simulink library "common_lib"  (R2021b)
settings: Solver=ode45  StartTime=0.0  StopTime=10.0  RelTol=1e-3
undefined symbols (not defined in the file or in its folder): ACCEL_PRE_MULT, C_C1GearNumbers, C_C1GearRatios, C_Calibration, C_DitherWaveform, C_GearOffset, C_GearRatioIn, C_GearRatioInverseOut, C_GearRatioOut, CLUTCH_INNER_LOOP_UPDATE_RATE, CONSTANT, DEGRADED_MODE_SIZE, Dem_EventStatusType, DiscIntNeverNeededParam, F_FAULT_ENUM, F_NOFAULT, F_OUTOFRANGE, F_RATELIMIT, FALSE, FMI14_SPECIAL_INSTRUCTIONS, FMI20_DATA_DRIFTED_HIGH, FMI21_DATA_DRIFTED_LOW, FMI29_RESERVED_FOR_SAE_ASSIGNMENT, FMI30_RESERVED_FOR_SAE_ASSIGNMENT, FMI31_CONDITION_EXISTS, FMI32_NO_FAULT, IC, k_accel, k_mean, LVDCU_OORH_FaultCntThd_C, MAX_UINT32, MEAN_PRE_MULT, NTriggers, QLTY_SIGNAL_FAILED, QLTY_SIGNAL_FULLY_FUNCTION, QLTY_SIGNAL_SUBSTITUTED_BY_1ST_CHOICE, QLTY_SIGNAL_SUBSTITUTED_BY_2ND_CHOICE, QLTY_SIGNAL_SUBSTITUTED_BY_3RD_CHOICE, QLTY_SIGNAL_SUBSTITUTED_BY_4TH_CHOICE, SAMPLE_TIME_100_mSec, SAMPLE_TIME_100_uSec, simin, T_TestPoint, TF_FALSE, TF_TRUE, TimeStep, TRUE, WORKSPACE_UPDATE_RATE, ZERO, Zero
libraries: $bdroot x120, simulink x27, simulink_extras x4, MBD_EPS_Local_Blockset x4
(part 9 of 10)

== system common_lib/Signal Conditioning/HydValveDither/CalculateActualFreq ==
  desired_freqency_hz : Inport
  sample_time : Inport  Port=2
  ClampAroundZero : $bdroot/Misc/ClampAroundZero  Tol=single(eps)
      settings: AttributesFormatString=tol=%<Tol>
  ClampAroundZero1 : $bdroot/Misc/ClampAroundZero  Tol=single(eps)
      settings: AttributesFormatString=tol=%<Tol>
  Constant4 : Constant  Value=single(0)
  Constant7 : Constant  Value=single(1)
  Constant8 : Constant  Value=single(1)
  Product4 : Product  RndMeth=Zero
  Product5 : Product  Inputs=*/  RndMeth=Zero
  Product6 : Product  RndMeth=Zero
  Product7 : Product  Inputs=*/  RndMeth=Zero
  Rounding Function : Rounding  Operator=round
  Switch : Switch  Criteria=u2 > Threshold
  realized_freq : Outport  VectorParamsAs1DForOutWhenUnconnected=off
  sample_times_per_cycle : Outport  Port=2  VectorParamsAs1DForOutWhenUnconnected=off
  wires:
  sample_time/1 -> Product4/1, Product6/1
  Constant7/1 -> Product5/1
  Product5/1 -> Rounding Function/1, sample_times_per_cycle/1  "sample_times_per_period"
  Rounding Function/1 -> Product6/2
  Constant8/1 -> Product7/1
  Product6/1 -> ClampAroundZero1/1
  desired_freqency_hz/1 -> Product4/2, Switch/2
  Product4/1 -> ClampAroundZero/1
  ClampAroundZero/1 -> Product5/2
  ClampAroundZero1/1 -> Product7/2
  Product7/1 -> Switch/1
  Switch/1 -> realized_freq/1
  Constant4/1 -> Switch/3

== system common_lib/Signal Conditioning/HydValveDither/TableBasedSignalGen ==
  sample_times_per_cycle : Inport
  Constant1 : Constant  Value=single(32768)
  Constant5 : Constant  Value=int32(1)
  Constant6 : Constant  Value=length(DitherWaveform)-1  OutDataTypeStr=uint16
  Constant9 : Constant  Value=length(DitherWaveform)-1  OutDataTypeStr=single
  Data Type Conversion2 : DataTypeConversion  OutDataTypeStr=uint16  RndMeth=Nearest
  Data Type Conversion3 : DataTypeConversion  OutDataTypeStr=int32  RndMeth=Nearest
  Direct Lookup Table (n-D) : LookupNDDirect  NumberOfTableDimensions=1  Table=DitherWaveform
  Discrete-Time Integrator : DiscreteIntegrator  IntegratorMethod=Accumulation: Forward Euler  ExternalReset=rising  SampleTime=ts  ShowStatePort=on  ICPrevOutput=DiscIntNeverNeededParam  ICPrevScaledInput=DiscIntNeverNeededParam
  MinMax : MinMax  Inputs=2
  MinMax1 : MinMax  Inputs=2
  Product8 : Product  Inputs=*/*  RndMeth=Zero
  Relational Operator : RelationalOperator  Operator=<=  OutDataTypeStr=boolean  RndMeth=Nearest
  out : Outport  VectorParamsAs1DForOutWhenUnconnected=off
  wires:
  Discrete-Time Integrator/1 -> Product8/1
  Relational Operator/1 -> [reset_integrator]
  [reset_integrator] -> Discrete-Time Integrator/2
  Product8/1 -> Data Type Conversion2/1
  Discrete-Time Integrator/State -> Relational Operator/2
  Constant5/1 -> Discrete-Time Integrator/1
  Data Type Conversion3/1 -> Relational Operator/1
  Constant9/1 -> Product8/3
  Constant6/1 -> MinMax/2
  Data Type Conversion2/1 -> MinMax/1
  MinMax/1 -> Direct Lookup Table (n-D)/1
  Direct Lookup Table (n-D)/1 -> out/1
  sample_times_per_cycle/1 -> Product8/2, MinMax1/2
  MinMax1/1 -> Data Type Conversion3/1
  Constant1/1 -> MinMax1/1

== system common_lib/Signal Conditioning/Obsolete Signal Conditioning/BooleanToTernary ==
  note: Boolean to Ternary Conversion
      | Eaton Corporation
  Boolean : Inport
  Constant1 : Constant  Value=TF_TRUE
  Constant4 : Constant  Value=TF_FALSE
  Switch : Switch  Threshold=0.5  ZeroCross=off
  Ternary : Outport  VectorParamsAs1DForOutWhenUnconnected=off
  wires:
  Boolean/1 -> Switch/2
  Switch/1 -> Ternary/1
  Constant4/1 -> Switch/3
  Constant1/1 -> Switch/1

== system common_lib/Signal Conditioning/Obsolete Signal Conditioning/Ternary To Boolean (Default False) ==
  note: Ternary To Boolean Conversion (Default False)
      | Eaton Corporation
  note: Outputs a FALSE upon an invalid or FALSE input
      | Outputs a TRUE upon a TRUE (149) input
  Ternary : Inport
  Constant1 : Constant  Value=TF_TRUE
  Data Type Conversion : DataTypeConversion  OutDataTypeStr=uint8  RndMeth=Zero
  Relational Operator : RelationalOperator  Operator===  ZeroCross=off  RndMeth=Nearest
  Boolean : Outport  VectorParamsAs1DForOutWhenUnconnected=off
  wires:
  Ternary/1 -> Data Type Conversion/1
  Relational Operator/1 -> Boolean/1
  Constant1/1 -> Relational Operator/1
  Data Type Conversion/1 -> Relational Operator/2

== system common_lib/Signal Conditioning/Obsolete Signal Conditioning/Ternary To Boolean (Default True) ==
  note: Outputs a TRUE upon an invalid or TRUE input
      | Outputs a FALSE upon a FALSE (89) input
  note: Ternary To Boolean Conversion (Default True)
      | Eaton Corporation
  Ternary : Inport
  Constant1 : Constant  Value=TF_FALSE
  Data Type Conversion : DataTypeConversion  OutDataTypeStr=uint8  RndMeth=Zero
  Relational Operator : RelationalOperator  Operator=~=  ZeroCross=off  RndMeth=Nearest
  Boolean : Outport  VectorParamsAs1DForOutWhenUnconnected=off
  wires:
  Data Type Conversion/1 -> Relational Operator/2
  Constant1/1 -> Relational Operator/1
  Relational Operator/1 -> Boolean/1
  Ternary/1 -> Data Type Conversion/1

== system common_lib/Signal Generators/Clu_2_1_3_1_1_1_TestSignalBuilder/TestFrequencyRamp ==
  TestFreqRampStartFreq : Inport
  TestFreqRampEndFreq : Inport  Port=2
  TestFreqRampTime : Inport  Port=3
  TestSignalEnable : Inport  Port=4
  Test_Reset : Inport  Port=5
  ClampAroundZero2 : $bdroot/Misc/ClampAroundZero  Tol=single(eps(1))
      settings: AttributesFormatString=tol=%<Tol>
  Constant1 : Constant  Value=CLUTCH_INNER_LOOP_UPDATE_RATE
  Constant3 : Constant  Value=ZERO
  Constant30 : Constant  Value=ZERO
  Constant4 : Constant  Value=ZERO
  Data Type Conversion : DataTypeConversion  OutDataTypeStr=single  RndMeth=Zero
  Integrator2 : $bdroot/Ctrl/Integrator  TimeStep=CLUTCH_INNER_LOOP_UPDATE_RATE  IC=single(0.0)
  Product6 : Product  Inputs=*/*  InputSameDT=on  OutDataTypeStr=Inherit: Same as first input
  Sum3 : Sum  Inputs=+-|  InputSameDT=on  OutDataTypeStr=Inherit: Same as first input
  Sum5 : Sum  Inputs=|++  InputSameDT=on  OutDataTypeStr=Inherit: Same as first input
  Switch1 : Switch  Threshold=0.5  ZeroCross=off
  TestFreqRampFreq : Outport  InitialOutput=[single(0)]  VectorParamsAs1DForOutWhenUnconnected=off
      settings: AttributesFormatString=InitialOutput=%<InitialOutput>\nOutputWhenDisabled=%<OutputWhenDisabled>
  wires:
  TestFreqRampEndFreq/1 -> Sum3/1, [TgtFreq]
  TestFreqRampStartFreq/1 -> Sum3/2, [InitFreq]
  Sum3/1 -> Product6/1
  TestFreqRampTime/1 -> ClampAroundZero2/1
  Constant30/1 -> Integrator2/4
  [TgtFreq] -> Integrator2/2
  Constant4/1 -> Integrator2/3
  Integrator2/1 -> Sum5/1
  Sum5/1 -> TestFreqRampFreq/1  "TestFreqRampFreq"
  [InitFreq] -> Sum5/2
  Switch1/1 -> Integrator2/1
  Product6/1 -> Switch1/1
  Constant3/1 -> Switch1/3
  ClampAroundZero2/1 -> Product6/2
  TestSignalEnable/1 -> Switch1/2
  Test_Reset/1 -> Integrator2/5
  Constant1/1 -> Data Type Conversion/1
  Data Type Conversion/1 -> Product6/3

== system common_lib/Signal Generators/Clu_2_1_3_1_1_1_TestSignalBuilder/TestOffsetRamp ==
  TestWaveOffsetRampStart : Inport
  TestWaveOffsetRampEnd : Inport  Port=2
  TestWaveOffsetRampTime : Inport  Port=3
  Test_Enable : Inport  Port=4
  Test_Reset : Inport  Port=5
  ClampAroundZero1 : $bdroot/Misc/ClampAroundZero  Tol=single(eps(1))
      settings: AttributesFormatString=tol=%<Tol>
  Constant11 : Constant  Value=ZERO
  Constant8 : Constant  Value=ZERO
  Constant9 : Constant  Value=ZERO
  Integrator3 : $bdroot/Ctrl/Integrator  TimeStep=CLUTCH_INNER_LOOP_UPDATE_RATE  IC=single(0.0)
  Product4 : Product  Inputs=*/  InputSameDT=on  OutDataTypeStr=Inherit: Same as first input
  Sum7 : Sum  Inputs=+-|  InputSameDT=on  OutDataTypeStr=Inherit: Same as first input
  Switch3 : Switch  Threshold=0.5  ZeroCross=off
  TestConstant : Outport  InitialOutput=[single(0)]  VectorParamsAs1DForOutWhenUnconnected=off
      settings: AttributesFormatString=InitialOutput=%<InitialOutput>\nOutputWhenDisabled=%<OutputWhenDisabled>
  TestOffsetRamp : Outport  Port=2  InitialOutput=[single(0)]  VectorParamsAs1DForOutWhenUnconnected=off
      settings: AttributesFormatString=InitialOutput=%<InitialOutput>\nOutputWhenDisabled=%<OutputWhenDisabled>
  wires:
  TestWaveOffsetRampStart/1 -> Sum7/2
  Sum7/1 -> Product4/1
  TestWaveOffsetRampTime/1 -> ClampAroundZero1/1
  Constant9/1 -> Integrator3/4
  [TestWaveOffsetRampEnd] -> Integrator3/2
  Constant11/1 -> Integrator3/3
  Switch3/1 -> Integrator3/1
  Product4/1 -> Switch3/1
  Constant8/1 -> Switch3/3
  ClampAroundZero1/1 -> Product4/2
  Integrator3/1 -> TestOffsetRamp/1
  TestWaveOffsetRampEnd/1 -> Sum7/1, [TestWaveOffsetRampEnd], TestConstant/1
  Test_Enable/1 -> Switch3/2
  Test_Reset/1 -> Integrator3/5

== system common_lib/Signal Generators/Clu_2_1_3_1_1_1_TestSignalBuilder/TestRampWaves ==
  TestOffsetRamp : Inport
  TestWave : Inport  Port=2
  TestWaveSignSwitch : Inport  Port=3
  Constant : Constant  Value=single(0.0)  SampleTime=-1
  EdgeTriggered Pulse : $bdroot/Misc/EdgeTriggered Pulse  Edge=FALSE to TRUE  Width=single(CLUTCH_INNER_LOOP_UPDATE_RATE)  Pulse=TRUE  TimeStep=CLUTCH_INNER_LOOP_UPDATE_RATE  Init=0
  Hold : $bdroot/Misc/Hold  SystemSampleTime=-1  VariantActivationTime=update diagram  Latency=0  AutoFrameSizeCalculation=off
  Relational Operator : RelationalOperator  Operator=>  ZeroCross=off  RndMeth=Nearest
  Sum1 : Sum  InputSameDT=on  OutDataTypeStr=Inherit: Same as first input
  Sum2 : Sum  InputSameDT=on  OutDataTypeStr=Inherit: Same as first input
  SineWave : Outport  VectorParamsAs1DForOutWhenUnconnected=off
  SquareWave : Outport  Port=2  VectorParamsAs1DForOutWhenUnconnected=off
  wires:
  Sum1/1 -> SineWave/1
  TestOffsetRamp/1 -> Hold/1, Sum1/1
  TestWave/1 -> Sum1/2, Sum2/2
  TestWaveSignSwitch/1 -> Relational Operator/1
  EdgeTriggered Pulse/1 -> Hold/Enable
  Hold/1 -> Sum2/1
  Sum2/1 -> SquareWave/1
  Relational Operator/1 -> EdgeTriggered Pulse/1
  Constant/1 -> Relational Operator/2

== system common_lib/Signal Generators/Clu_2_1_3_1_1_1_TestSignalBuilder/TestWaveCreation ==
  note: Outputtype
      | 0. Constant
      | 1. Ramp
      | 2. Sine Wave
      | 3. Square Wave
      | 4. Zero
  TestFreqRampFreq : Inport
  TestWaveAmplitude : Inport  Port=2
  Test_Reset : Inport  Port=3
  CluPresCmdTestSignalType : Inport  Port=4
  Constant1 : Constant  Value=-1
  Constant10 : Constant  Value=pi/2.0
  Constant12 : Constant  Value=-1.0
  Constant13 : Constant  Value=1.0
  Constant2 : Constant  Value=single(0.0)
  Constant3 : Constant  Value=single(0.0)
  Constant30 : Constant  Value=ZERO
  Constant4 : Constant  Value=single(0.0)
  Data Type Conversion{12..13,19..20} (4 alike) : DataTypeConversion  OutDataTypeStr=single  RndMeth=Zero
  Integrator1 : $bdroot/Ctrl/Integrator  TimeStep=CLUTCH_INNER_LOOP_UPDATE_RATE  IC=single(0.0)
  Multiport Switch : MultiPortSwitch  DataPortOrder=Zero-based contiguous  Inputs=4  DataPortForDefault=Additional data port  zeroidx=on
  Product1 : Product  Inputs=**  InputSameDT=on  OutDataTypeStr=Inherit: Same as first input
  Product2 : Product  Inputs=**  InputSameDT=on  OutDataTypeStr=Inherit: Same as first input
  Product5 : Product  Inputs=**  InputSameDT=on  OutDataTypeStr=Inherit: Same as first input
  Relay : $bdroot/Slink/Relay  init=single(1.0)
  Sine1 : $bdroot/Misc/Sine
  Unit Delay4 : UnitDelay  InitialCondition=single(1.0)  SampleTime=-1  HasFrameUpgradeWarning=on
      settings: AttributesFormatString=ic=%<X0>
  TestWave : Outport  InitialOutput=[single(0)]  VectorParamsAs1DForOutWhenUnconnected=off
      settings: AttributesFormatString=InitialOutput=%<InitialOutput>\nOutputWhenDisabled=%<OutputWhenDisabled>
  TestWaveSignSwitch : Outport  Port=2  InitialOutput=[single(0)]  VectorParamsAs1DForOutWhenUnconnected=off
      settings: AttributesFormatString=InitialOutput=%<InitialOutput>\nOutputWhenDisabled=%<OutputWhenDisabled>
  wires:
  Constant12/1 -> Data Type Conversion19/1
  Constant13/1 -> Data Type Conversion20/1
  Data Type Conversion19/1 -> Relay/4
  Data Type Conversion20/1 -> Relay/5
  Relay/1 -> Unit Delay4/1, Multiport Switch/5, TestWaveSignSwitch/1
  Unit Delay4/1 -> [TestWaveSignSwitch]
  Integrator1/1 -> Relay/1, Sine1/1
  TestWaveAmplitude/1 -> Product2/1
  Product2/1 -> TestWave/1
  [TestWaveSignSwitch] -> Product5/2
  Product5/1 -> Integrator1/1  "ChirpFrequency"
  Constant10/1 -> Data Type Conversion12/1, Product1/1
  Product1/1 -> Data Type Conversion13/1
  Constant1/1 -> Product1/2
  Data Type Conversion12/1 -> Integrator1/2, Relay/2
  Data Type Conversion13/1 -> Integrator1/3, Relay/3
  Constant30/1 -> Integrator1/4
  Test_Reset/1 -> Integrator1/5
  TestFreqRampFreq/1 -> Product5/1
  CluPresCmdTestSignalType/1 -> Multiport Switch/1
  Constant2/1 -> Multiport Switch/2
  Constant3/1 -> Multiport Switch/3
  Constant4/1 -> Multiport Switch/6
  Multiport Switch/1 -> Product2/2
  Sine1/1 -> Multiport Switch/4

== system common_lib/Signal Generators/Signal Generator Components/TestSignalPeriod ==
  TestSignalFrequency : Inport
  ClampAboveZero : $bdroot/Misc/ClampAboveZero  Tol=single(0.0001)
      settings: AttributesFormatString=tol=%<Tol>
  ClampAroundZero1 : $bdroot/Misc/ClampAroundZero  Tol=single(0.01)
      settings: AttributesFormatString=tol=%<Tol>
  Constant1 : Constant  Value=TimeStep  SampleTime=-1
  Constant35 : Constant  Value=single(2.0)  SampleTime=-1
  Constant39 : Constant  Value=single(1.0)  SampleTime=-1
  Data Type Conversion1 : DataTypeConversion  OutDataTypeStr=single
  MinMax1 : MinMax  Function=max  Inputs=2  InputSameDT=on  ZeroCross=off
  Product15 : Product  Inputs=*/  OutDataTypeStr=Inherit: Same as first input
  Product19 : Product  Inputs=**  InputSameDT=on  OutDataTypeStr=Inherit: Same as first input
  TestSignalPeriod : Outport  VectorParamsAs1DForOutWhenUnconnected=off
  wires:
  Product15/1 -> MinMax1/1
  Constant39/1 -> Product15/1
  ClampAroundZero1/1 -> Product15/2
  TestSignalFrequency/1 -> ClampAroundZero1/1
  Constant1/1 -> Data Type Conversion1/1
  Constant35/1 -> Product19/2
  Product19/1 -> MinMax1/2
  MinMax1/1 -> TestSignalPeriod/1  "TestSignalPeriod"
  ClampAboveZero/1 -> Product19/1
  Data Type Conversion1/1 -> ClampAboveZero/1

== system common_lib/Signal Generators/Signal Generator Components/TestSignalPeriodTimer ==
  TestSignalReset : Inport
  TestSignalPeriod : Inport  Port=2
  ClampAboveZero : $bdroot/Misc/ClampAboveZero  Tol=single(0.0001)
      settings: AttributesFormatString=tol=%<Tol>
  Constant1 : Constant  Value=TimeStep  SampleTime=-1
  Constant40 : Constant  Value=false  SampleTime=-1
  Constant41 : Constant  Value=single(0.0)
  Data Type Conversion7 : DataTypeConversion  OutDataTypeStr=single
  Logical Operator1 : Logic  Operator=OR  Inputs=3  AllPortsSameDT=off
  Relational Operator4 : RelationalOperator  ZeroCross=off  RndMeth=Nearest
  Sum5 : Sum  Inputs=2
  Switch5 : Switch  Threshold=0.5  ZeroCross=off
  Unit Delay4 : UnitDelay  InitialCondition=true  SampleTime=-1  HasFrameUpgradeWarning=on
      settings: AttributesFormatString=ic=%<X0>
  Unit Delay5 : UnitDelay  InitialCondition=single(0.0)  SampleTime=-1  HasFrameUpgradeWarning=on
      settings: AttributesFormatString=ic=%<X0>
  TestSignalTime : Outport  VectorParamsAs1DForOutWhenUnconnected=off
  wires:
  TestSignalReset/1 -> Logical Operator1/2
  Logical Operator1/1 -> Switch5/2
  Switch5/1 -> Unit Delay5/1, TestSignalTime/1  "TestSignalTime"
  Sum5/1 -> Switch5/3
  Constant41/1 -> Switch5/1
  Unit Delay4/1 -> Logical Operator1/1
  Constant40/1 -> Unit Delay4/1
  TestSignalPeriod/1 -> Relational Operator4/2
  Relational Operator4/1 -> Logical Operator1/3
  Unit Delay5/1 -> Relational Operator4/1, Sum5/1
  Constant1/1 -> Data Type Conversion7/1
  Data Type Conversion7/1 -> ClampAboveZero/1
  ClampAboveZero/1 -> Sum5/2

== system common_lib/Signal Generators/Signal Generator Components/TestSignalRamp ==
  TestSignalRampStart : Inport
  TestSignalRampEnd : Inport  Port=2
  TestSignalRampTime : Inport  Port=3
  TestSignalReset : Inport  Port=4
  Abs : Abs  ZeroCross=off
  Constant35 : Constant  Value=single(0.01)  SampleTime=-1
  Logical Operator : Logic  AllPortsSameDT=off
  Logical Operator1 : Logic  Operator=NOT  AllPortsSameDT=off
  Logical Operator2 : Logic  Operator=NOT  AllPortsSameDT=off
  Logical Operator3 : Logic  Operator=OR  AllPortsSameDT=off
  Relational Operator : RelationalOperator  ZeroCross=off  RndMeth=Nearest
  Sum : Sum  Inputs=+-
  TestSignalRampEnabled : Subsystem
  Unit Delay : UnitDelay  InitialCondition=CLUTCH_INNER_LOOP_UPDATE_RATE  SampleTime=-1  HasFrameUpgradeWarning=on
      settings: AttributesFormatString=ic=%<X0>
  TestSignal : Outport  VectorParamsAs1DForOutWhenUnconnected=off
  wires:
  Logical Operator3/1 -> Logical Operator/2
  Logical Operator2/1 -> Logical Operator3/2
  Unit Delay/1 -> Logical Operator2/1
  Logical Operator1/1 -> Logical Operator3/1
  Logical Operator/1 -> TestSignalRampEnabled/Enable
  Relational Operator/1 -> Logical Operator/1
  Constant35/1 -> Relational Operator/2
  Abs/1 -> Relational Operator/1
  Sum/1 -> Abs/1
  TestSignalRampTime/1 -> TestSignalRampEnabled/3(TestSignalFreqRampTime)
  TestSignalRampEnabled/1(TestSignalFrequency) -> TestSignal/1
  TestSignalRampEnd/1 -> Sum/2, TestSignalRampEnabled/2(TestSignalFreqRampEnd)
  TestSignalRampStart/1 -> Sum/1, TestSignalRampEnabled/1(TestSignalFrequencyIn)
  TestSignalReset/1 -> Unit Delay/1, Logical Operator1/1, TestSignalRampEnabled/4(TestSignalReset)

== system common_lib/Signal Generators/Signal Generator Components/TestSignalSineWave ==
  TestSignalPk2PkAmplitude : Inport
  TestSignalOffset : Inport  Port=2
  TestSignalTime : Inport  Port=3
  TestSignalPeriod : Inport  Port=4
  TestSignalReset : Inport  Port=5
  Constant1 : Constant  Value=single(0.0)
  Data Type Conversion4 : DataTypeConversion  OutDataTypeStr=uint32  RndMeth=Zero
  Look-Up Table : Lookup  InputValues=single([0 0.25 0.5 0.75 1])  Table=single([0 pi/2 0 -pi/2 0])  LookUpMeth=Interpolation-Use End Values
      settings: AttributesFormatString=X=%<InputValues>\nY= %<OutputValues>
  Product1 : Product  Inputs=*/  OutDataTypeStr=Inherit: Same as first input
  Product16 : Product  Inputs=*/  OutDataTypeStr=Inherit: Same as first input
  Product18 : Product  Inputs=**  OutDataTypeStr=Inherit: Same as first input
  Sine1 : $bdroot/Misc/Sine
  Sum3 : Sum  Inputs=+-
  Sum4 : Sum
  Switch1 : Switch  Threshold=0.5  ZeroCross=off
  TestSignal : Outport  VectorParamsAs1DForOutWhenUnconnected=off
  wires:
  Sine1/1 -> Product18/1
  Look-Up Table/1 -> Sine1/1
  Product1/1 -> Look-Up Table/1  "TestSignalPeriodFrac"
  [TestSignalPeriod] -> Product1/2
  Switch1/1 -> Sum4/1
  Constant1/1 -> Switch1/1
  TestSignalReset/1 -> Switch1/2
  TestSignalPk2PkAmplitude/1 -> Product18/2
  TestSignalOffset/1 -> Sum4/2
  Sum4/1 -> TestSignal/1  "TestSignal"
  Product16/1 -> Sum3/1, Data Type Conversion4/1
  Data Type Conversion4/1 -> Sum3/2
  Sum3/1 -> Product1/1
  Product18/1 -> Switch1/3
  TestSignalTime/1 -> Product16/1, [TestSignalTime]
  TestSignalPeriod/1 -> Product16/2, [TestSignalPeriod]

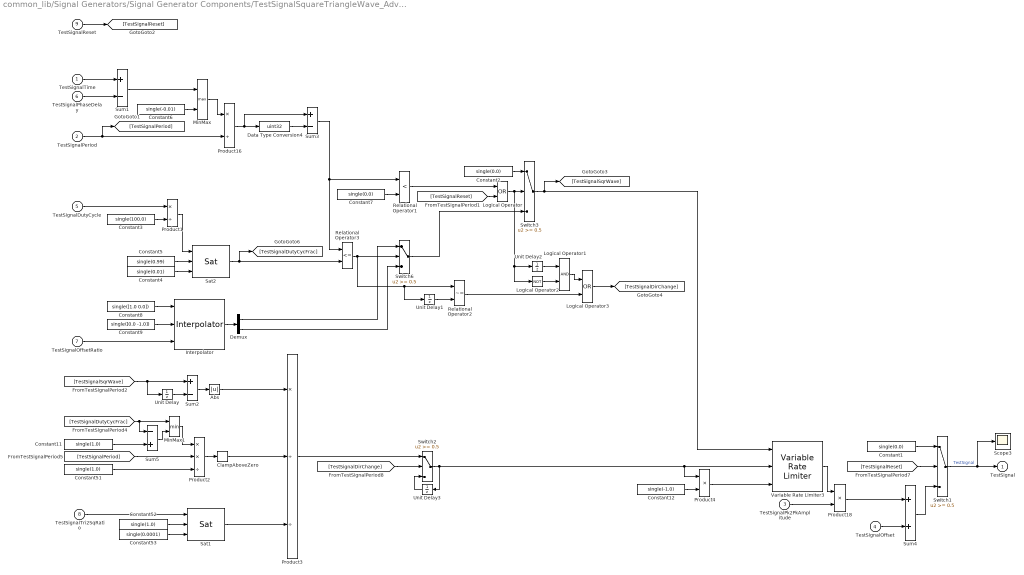
== system common_lib/Signal Generators/Signal Generator Components/TestSignalSquareTriangleWave_Advanced ==
  TestSignalTime : Inport
  TestSignalPeriod : Inport  Port=2
  TestSignalPk2PkAmplitude : Inport  Port=3
  TestSignalOffset : Inport  Port=4
  TestSignalDutyCycle : Inport  Port=5
  TestSignalPhaseDelay : Inport  Port=6
  TestSignalOffsetRatio : Inport  Port=7
  TestSignalTri2SqRatio : Inport  Port=8
  TestSignalReset : Inport  Port=9
  Abs : Abs  ZeroCross=off
  ClampAboveZero : $bdroot/Misc/ClampAboveZero  Tol=single(0.001)
      settings: AttributesFormatString=tol=%<Tol>
  Constant1 : Constant  Value=single(0.0)
  Constant11 : Constant  Value=single(1.0)
  Constant12 : Constant  Value=single(-1.0)
  Constant2 : Constant  Value=single(0.0)
  Constant3 : Constant  Value=single(100.0)
  Constant4 : Constant  Value=single(0.01)
  Constant5 : Constant  Value=single(0.99)
  Constant51 : Constant  Value=single(1.0)
  Constant52 : Constant  Value=single(1.0)
  Constant53 : Constant  Value=single(0.0001)
  Constant6 : Constant  Value=single(-0.01)
  Constant7 : Constant  Value=single(0.0)
  Constant8 : Constant  Value=single([1.0 0.0])
  Constant9 : Constant  Value=single([0.0 -1.0])
  Data Type Conversion4 : DataTypeConversion  OutDataTypeStr=uint32  RndMeth=Zero
  Demux : Demux  Outputs=2
  Interpolator : $bdroot/Tbl/Interpolator  DType=Single
  Logical Operator : Logic  Operator=OR  AllPortsSameDT=off
  Logical Operator1 : Logic  AllPortsSameDT=off
  Logical Operator2 : Logic  Operator=NOT  AllPortsSameDT=off
  Logical Operator3 : Logic  Operator=OR  AllPortsSameDT=off
  MinMax : MinMax  Function=max  Inputs=2  InputSameDT=on  ZeroCross=off
  MinMax1 : MinMax  Inputs=2  InputSameDT=on  ZeroCross=off
  Product1 : Product  Inputs=*/  OutDataTypeStr=Inherit: Same as first input
  Product16 : Product  Inputs=*/  OutDataTypeStr=Inherit: Same as first input
  Product18 : Product  Inputs=**  OutDataTypeStr=Inherit: Same as first input
  Product2 : Product  Inputs=**/  OutDataTypeStr=Inherit: Same as first input
  Product3 : Product  Inputs=*//  OutDataTypeStr=Inherit: Same as first input
  Product4 : Product  Inputs=**  OutDataTypeStr=Inherit: Same as first input
  Relational Operator1 : RelationalOperator  Operator=<  ZeroCross=off  RndMeth=Nearest
  Relational Operator2 : RelationalOperator  Operator=~=  ZeroCross=off  RndMeth=Nearest
  Relational Operator3 : RelationalOperator  Operator=<=  ZeroCross=off  RndMeth=Nearest
  Sat1 : $bdroot/Slink/Sat
  Sat2 : $bdroot/Slink/Sat
  Scope3 : Scope
  Sum1 : Sum  Inputs=+-
  Sum2 : Sum  Inputs=+-
  Sum3 : Sum  Inputs=+-
  Sum4 : Sum
  Sum5 : Sum  Inputs=-+
  Switch{1..3,6} (4 alike) : Switch  Threshold=0.5  ZeroCross=off
  Unit Delay : UnitDelay  InitialCondition=single(0.0)  SampleTime=-1  HasFrameUpgradeWarning=on
      settings: AttributesFormatString=ic=%<X0>
  Unit Delay1 : UnitDelay  InitialCondition=false  SampleTime=-1  HasFrameUpgradeWarning=on
      settings: AttributesFormatString=ic=%<X0>
  Unit Delay2 : UnitDelay  InitialCondition=false  SampleTime=-1  HasFrameUpgradeWarning=on
      settings: AttributesFormatString=ic=%<X0>
  Unit Delay3 : UnitDelay  InitialCondition=single(0.0)  SampleTime=-1  HasFrameUpgradeWarning=on
      settings: AttributesFormatString=ic=%<X0>
  Variable Rate Limiter3 : $bdroot/Slink/Variable Rate Limiter  TimeStep=TimeStep  ic=single(0.0)
  TestSignal : Outport  VectorParamsAs1DForOutWhenUnconnected=off
  wires:
  MinMax1/1 -> Product2/1
  Product4/1 -> Variable Rate Limiter3/3
  Constant12/1 -> Product4/2
  Abs/1 -> Product3/1
  [TestSignalDirChange] -> Switch2/2
  Unit Delay3/1 -> Switch2/3
  Switch2/1 -> Unit Delay3/1, Product4/1, Variable Rate Limiter3/2
  [TestSignalReset] -> Switch1/2
  Product3/1 -> Switch2/1
  Sum5/1 -> MinMax1/2
  Constant11/1 -> Sum5/2
  ClampAboveZero/1 -> Product3/2
  Sum2/1 -> Abs/1
  Product2/1 -> ClampAboveZero/1
  [TestSignalPeriod] -> Product2/2
  [TestSignalDutyCycFrac] -> MinMax1/1, Sum5/1
  Unit Delay/1 -> Sum2/2
  Logical Operator3/1 -> [TestSignalDirChange]
  Relational Operator2/1 -> Logical Operator3/2
  Logical Operator1/1 -> Logical Operator3/1
  Logical Operator2/1 -> Logical Operator1/2
  Unit Delay2/1 -> Logical Operator1/1
  Unit Delay1/1 -> Relational Operator2/2
  [TestSignalSqrWave] -> Sum2/1, Unit Delay/1
  Logical Operator/1 -> Logical Operator2/1, Unit Delay2/1, Switch3/2
  [TestSignalReset] -> Logical Operator/2
  Demux/2 -> Switch6/3
  Demux/1 -> Switch6/1
  Interpolator/1 -> Demux/1
  Constant2/1 -> Switch3/1
  Constant8/1 -> Interpolator/1
  Switch3/1 -> [TestSignalSqrWave], Variable Rate Limiter3/1
  Constant9/1 -> Interpolator/2
  TestSignalOffsetRatio/1 -> Interpolator/3
  Relational Operator1/1 -> Logical Operator/1
  Constant7/1 -> Relational Operator1/2
  MinMax/1 -> Product16/1
  Constant6/1 -> MinMax/2
  TestSignalPhaseDelay/1 -> Sum1/2
  Sum1/1 -> MinMax/1
  Sat2/1 -> [TestSignalDutyCycFrac], Relational Operator3/2
  Constant5/1 -> Sat2/2
  Constant4/1 -> Sat2/3
  Product1/1 -> Sat2/1
  Constant3/1 -> Product1/2
  TestSignalDutyCycle/1 -> Product1/1
  Switch1/1 -> Scope3/1, TestSignal/1  "TestSignal"
  Constant1/1 -> Switch1/1
  Sat1/1 -> Product3/3
  Constant53/1 -> Sat1/3
  Constant52/1 -> Sat1/2
  TestSignalTri2SqRatio/1 -> Sat1/1
  Constant51/1 -> Product2/3
  Variable Rate Limiter3/1 -> Product18/1
  TestSignalPk2PkAmplitude/1 -> Product18/2
  TestSignalOffset/1 -> Sum4/2
  Product16/1 -> Sum3/1, Data Type Conversion4/1
  Data Type Conversion4/1 -> Sum3/2
  Sum3/1 -> Relational Operator1/1, Relational Operator3/1
  Relational Operator3/1 -> Unit Delay1/1, Relational Operator2/1, Switch6/2
  Switch6/1 -> Switch3/3
  Product18/1 -> Sum4/1
  TestSignalTime/1 -> Sum1/1
  TestSignalPeriod/1 -> Product16/2, [TestSignalPeriod]
  Sum4/1 -> Switch1/3
  TestSignalReset/1 -> [TestSignalReset]

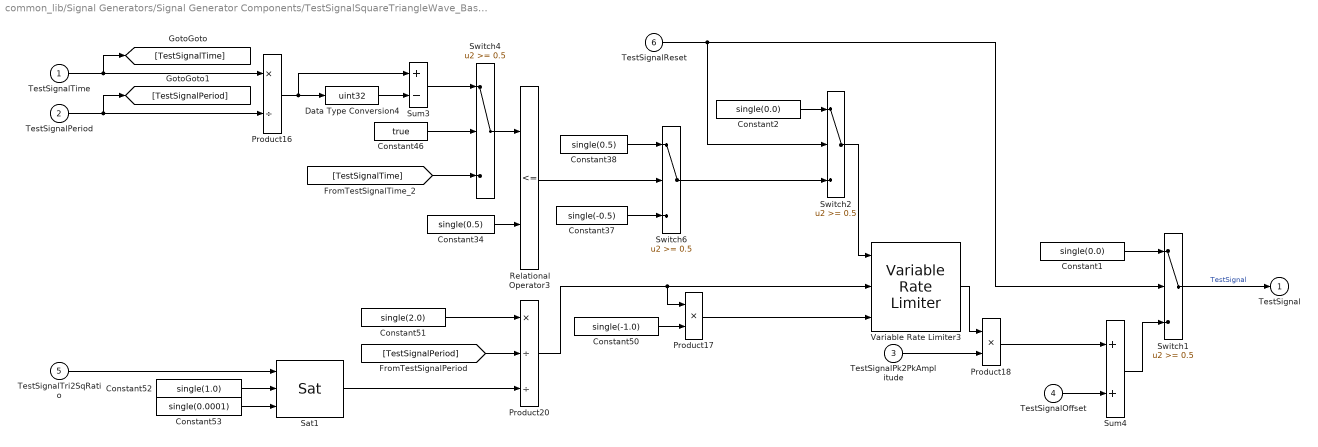
== system common_lib/Signal Generators/Signal Generator Components/TestSignalSquareTriangleWave_Basic ==
  TestSignalTime : Inport
  TestSignalPeriod : Inport  Port=2
  TestSignalPk2PkAmplitude : Inport  Port=3
  TestSignalOffset : Inport  Port=4
  TestSignalTri2SqRatio : Inport  Port=5
  TestSignalReset : Inport  Port=6
  Constant1 : Constant  Value=single(0.0)
  Constant2 : Constant  Value=single(0.0)
  Constant34 : Constant  Value=single(0.5)  SampleTime=-1
  Constant37 : Constant  Value=single(-0.5)  SampleTime=-1
  Constant38 : Constant  Value=single(0.5)  SampleTime=-1
  Constant46 : Constant  Value=true  SampleTime=-1
  Constant50 : Constant  Value=single(-1.0)
  Constant51 : Constant  Value=single(2.0)
  Constant52 : Constant  Value=single(1.0)
  Constant53 : Constant  Value=single(0.0001)
  Data Type Conversion4 : DataTypeConversion  OutDataTypeStr=uint32  RndMeth=Zero
  Product16 : Product  Inputs=*/  OutDataTypeStr=Inherit: Same as first input
  Product17 : Product  Inputs=**  OutDataTypeStr=Inherit: Same as first input
  Product18 : Product  Inputs=**  OutDataTypeStr=Inherit: Same as first input
  Product20 : Product  Inputs=*//  OutDataTypeStr=Inherit: Same as first input
  Relational Operator3 : RelationalOperator  Operator=<=  ZeroCross=off  RndMeth=Nearest
  Sat1 : $bdroot/Slink/Sat
  Sum3 : Sum  Inputs=+-
  Sum4 : Sum
  Switch{1..2,4,6} (4 alike) : Switch  Threshold=0.5  ZeroCross=off
  Variable Rate Limiter3 : $bdroot/Slink/Variable Rate Limiter  TimeStep=TimeStep  ic=single(0.0)
  TestSignal : Outport  VectorParamsAs1DForOutWhenUnconnected=off
  wires:
  Switch2/1 -> Variable Rate Limiter3/1
  Constant2/1 -> Switch2/1
  TestSignalReset/1 -> Switch1/2, Switch2/2
  Sum4/1 -> Switch1/3
  TestSignalPeriod/1 -> [TestSignalPeriod], Product16/2
  TestSignalTime/1 -> [TestSignalTime], Product16/1
  Product18/1 -> Sum4/1
  Switch6/1 -> Switch2/3
  Constant38/1 -> Switch6/1
  Constant37/1 -> Switch6/3
  Relational Operator3/1 -> Switch6/2
  Switch4/1 -> Relational Operator3/1
  [TestSignalTime] -> Switch4/3
  Constant46/1 -> Switch4/2
  Sum3/1 -> Switch4/1
  Data Type Conversion4/1 -> Sum3/2
  Product16/1 -> Data Type Conversion4/1, Sum3/1
  Constant34/1 -> Relational Operator3/2
  TestSignalOffset/1 -> Sum4/2
  TestSignalPk2PkAmplitude/1 -> Product18/2
  Product20/1 -> Product17/1, Variable Rate Limiter3/2
  Product17/1 -> Variable Rate Limiter3/3
  Constant50/1 -> Product17/2
  Variable Rate Limiter3/1 -> Product18/1
  Constant51/1 -> Product20/1
  [TestSignalPeriod] -> Product20/2
  TestSignalTri2SqRatio/1 -> Sat1/1
  Constant52/1 -> Sat1/2
  Constant53/1 -> Sat1/3
  Sat1/1 -> Product20/3
  Constant1/1 -> Switch1/1
  Switch1/1 -> TestSignal/1  "TestSignal"

== system common_lib/Signal Generators/Signal Generator Components/TestSignalTimer ==
  TestSignalReset : Inport
  Constant1 : Constant  Value=TimeStep  SampleTime=-1
  Constant40 : Constant  Value=false  SampleTime=-1
  Constant41 : Constant  Value=single(0.0)
  Constant43 : Constant  Value=single(1000000)
  Data Type Conversion7 : DataTypeConversion  OutDataTypeStr=single
  Logical Operator1 : Logic  Operator=OR  Inputs=3  AllPortsSameDT=off
  Relational Operator4 : RelationalOperator  ZeroCross=off  RndMeth=Nearest
  Sum5 : Sum  Inputs=2
  Switch5 : Switch  Threshold=0.5  ZeroCross=off
  Unit Delay4 : UnitDelay  InitialCondition=true  SampleTime=-1  HasFrameUpgradeWarning=on
      settings: AttributesFormatString=ic=%<X0>
  Unit Delay5 : UnitDelay  InitialCondition=single(0.0)  SampleTime=-1  HasFrameUpgradeWarning=on
      settings: AttributesFormatString=ic=%<X0>
  TestSignalTime : Outport  VectorParamsAs1DForOutWhenUnconnected=off
  wires:
  Constant1/1 -> Data Type Conversion7/1
  TestSignalReset/1 -> Logical Operator1/2
  Logical Operator1/1 -> Switch5/2
  Switch5/1 -> Unit Delay5/1, TestSignalTime/1  "TestSignalTime"
  Sum5/1 -> Switch5/3
  Constant41/1 -> Switch5/1
  Unit Delay4/1 -> Logical Operator1/1
  Constant40/1 -> Unit Delay4/1
  Constant43/1 -> Relational Operator4/2
  Relational Operator4/1 -> Logical Operator1/3
  Unit Delay5/1 -> Relational Operator4/1, Sum5/1
  Data Type Conversion7/1 -> Sum5/2

== system common_lib/Tbl/XY Interpolator1/XYInterp ==
  y_value_1 : Inport
  y_value_0 : Inport  Port=2
  x_value_1 : Inport  Port=3
  x_value_0 : Inport  Port=4
  x_value : Inport  Port=5
  ClampAroundZero : $bdroot/Misc/ClampAroundZero  Tol=Tol
  Constant1 : Constant  Value=Zero
  Constant2 : Constant  Value=One
  Product1 : Product  Inputs=*/  InputSameDT=on  OutDataTypeStr=Inherit: Same as first input
  Product2 : Product  Inputs=**  InputSameDT=on  OutDataTypeStr=Inherit: Same as first input
  Sat : $bdroot/Slink/Sat
  Sum : Sum  Inputs=+-  InputSameDT=on  OutDataTypeStr=Inherit: Same as first input
  Sum1 : Sum  Inputs=|++  InputSameDT=on  OutDataTypeStr=Inherit: Same as first input
  Sum2 : Sum  Inputs=-+  InputSameDT=on  OutDataTypeStr=Inherit: Same as first input
  Sum3 : Sum  Inputs=+-  InputSameDT=on  OutDataTypeStr=Inherit: Same as first input
  output : Outport  VectorParamsAs1DForOutWhenUnconnected=off
  wires:
  y_value_0/1 -> Sum1/2, Sum/2
  y_value_1/1 -> Sum/1
  Sum1/1 -> output/1
  Product2/1 -> Sum1/1
  Sum/1 -> Product2/1
  x_value/1 -> Sum3/1
  x_value_0/1 -> Sum3/2, Sum2/1
  Sum3/1 -> Product1/1
  x_value_1/1 -> Sum2/2
  Sum2/1 -> ClampAroundZero/1
  ClampAroundZero/1 -> Product1/2
  Product1/1 -> Sat/1
  Sat/1 -> Product2/2
  Constant2/1 -> Sat/2
  Constant1/1 -> Sat/3

== system common_lib/Ctrl/DTNA_PIgov/Integrator/Sat ==
  note: Common Library::Simulink Enhancements::Saturation
  input : Inport
  ulim : Inport  Port=2
  llim : Inport  Port=3
  MinMax : MinMax  Function=max  Inputs=2  InputSameDT=on  ZeroCross=off
  MinMax1 : MinMax  Inputs=2  InputSameDT=on  OutDataTypeStr=Inherit: Inherit via back propagation  ZeroCross=off
  output : Outport  VectorParamsAs1DForOutWhenUnconnected=off
  wires:
  MinMax/1 -> output/1
  llim/1 -> MinMax/2
  MinMax1/1 -> MinMax/1
  ulim/1 -> MinMax1/2
  input/1 -> MinMax1/1

== system common_lib/Diagnostics/Calibration Enabled MinMax OOR/Enabled OOR/OOR MinMax Capture ==
  Input : Inport
  Hold : Inport  Port=2
  Enable : EnablePort  ZeroCross=off
  CL MinMax Capture : $bdroot/Diag/CL MinMax Capture  CaptureType=Max  InDataType=single
  CL MinMax Capture1 : $bdroot/Diag/CL MinMax Capture  CaptureType=Min  InDataType=single
  DRDataStoreRead : DataStoreRead  DataStoreName=InitializeStates  IndexOptions=Index vector (dialog)  Indices=1  OutputSizes=1
  Max : Outport  VectorParamsAs1DForOutWhenUnconnected=off
  Min : Outport  Port=2  VectorParamsAs1DForOutWhenUnconnected=off
  wires:
  Input/1 -> CL MinMax Capture1/1, CL MinMax Capture/1
  Hold/1 -> CL MinMax Capture1/2, CL MinMax Capture/2
  DRDataStoreRead/1 -> CL MinMax Capture/3, CL MinMax Capture1/3
  CL MinMax Capture/1 -> Max/1
  CL MinMax Capture1/1 -> Min/1

== system common_lib/Diagnostics/Calibration Enabled MinMax RLim/Enabled RLim/RLim MinMax Capture ==
  Input : Inport
  Hold : Inport  Port=2
  Enable : EnablePort  ZeroCross=off
  CL MinMax Capture : $bdroot/Diag/CL MinMax Capture  CaptureType=Max  InDataType=single
  CL MinMax Capture1 : $bdroot/Diag/CL MinMax Capture  CaptureType=Min  InDataType=single
  DRDataStoreRead : DataStoreRead  DataStoreName=InitializeStates  IndexOptions=Index vector (dialog)  Indices=1  OutputSizes=1
  Sum1 : Sum  Inputs=|+-  InputSameDT=on  OutDataTypeStr=Inherit: Same as first input
  Unit Delay2 : UnitDelay  InitialCondition=Zero  SampleTime=-1  HasFrameUpgradeWarning=on
      settings: AttributesFormatString=ic=%<X0>
  Max : Outport  VectorParamsAs1DForOutWhenUnconnected=off
  Min : Outport  Port=2  VectorParamsAs1DForOutWhenUnconnected=off
  wires:
  Input/1 -> Sum1/1, Unit Delay2/1
  Hold/1 -> CL MinMax Capture1/2, CL MinMax Capture/2
  CL MinMax Capture/1 -> Max/1
  CL MinMax Capture1/1 -> Min/1
  Unit Delay2/1 -> Sum1/2
  Sum1/1 -> CL MinMax Capture1/1, CL MinMax Capture/1
  DRDataStoreRead/1 -> CL MinMax Capture/3, CL MinMax Capture1/3

== system common_lib/Diagnostics/Calibration Enabled MinMax RLim/Enabled RLim/RateLimit ==
  in : Inport
  rlim : Inport  Port=2
  ext_fault? : Inport  Port=3
  Constant2 : Constant  Value=TimeStep
  DRDataStoreRead : DataStoreRead  DataStoreName=InitializeStates  IndexOptions=Index vector (dialog)  Indices=1  OutputSizes=1
  Data Type Conversion : DataTypeConversion  OutDataTypeStr=single
  Logical Operator : Logic  Operator=NOT
  OOR Fault Detection : $bdroot/Diag/OOR Fault Detection  InitialValue=IC
  Product1 : Product  InputSameDT=on  OutDataTypeStr=Inherit: Same as first input
  Sum1 : Sum  Inputs=-+|  InputSameDT=on  OutDataTypeStr=Inherit: Same as first input
  Sum2 : Sum  Inputs=|++  InputSameDT=on  OutDataTypeStr=Inherit: Same as first input
  Sum3 : Sum  Inputs=++|  InputSameDT=on  OutDataTypeStr=Inherit: Same as first input
  Unit Delay : UnitDelay  InitialCondition=Zero  SampleTime=-1  HasFrameUpgradeWarning=on
      settings: AttributesFormatString=ic=%<X0>
  Unit Delay1 : UnitDelay  InitialCondition=false  SampleTime=-1  HasFrameUpgradeWarning=on
      settings: AttributesFormatString=ic=%<X0>
  Unit Delay2 : UnitDelay  InitialCondition=Zero  SampleTime=-1  HasFrameUpgradeWarning=on
      settings: AttributesFormatString=ic=%<X0>
  inc switch : Switch  Threshold=0.5  ZeroCross=off  InputSameDT=on
  inc switch1 : Switch  Threshold=0.5  ZeroCross=off  InputSameDT=on
  out : Outport  VectorParamsAs1DForOutWhenUnconnected=off
  fault? : Outport  Port=2  VectorParamsAs1DForOutWhenUnconnected=off
  wires:
  Constant2/1 -> Data Type Conversion/1
  Data Type Conversion/1 -> Product1/1
  inc switch1/1 -> Sum2/1, Sum1/2
  Unit Delay/1 -> inc switch1/1
  Unit Delay1/1 -> inc switch/2
  Unit Delay2/1 -> Sum3/1
  Sum3/1 -> inc switch/1
  Product1/1 -> Sum3/2, inc switch/3
  rlim/1 -> Product1/2
  inc switch/1 -> Unit Delay2/1, Sum1/1, Sum2/2
  Sum2/1 -> OOR Fault Detection/2
  Sum1/1 -> OOR Fault Detection/3
  OOR Fault Detection/2 -> Unit Delay1/1, fault?/1
  OOR Fault Detection/1 -> Unit Delay/1, out/1
  ext_fault?/1 -> OOR Fault Detection/4
  in/1 -> inc switch1/3, OOR Fault Detection/1
  DRDataStoreRead/1 -> Logical Operator/1
  Logical Operator/1 -> inc switch1/2

== system common_lib/Diagnostics/DTNA_Diag/CC_Diag/Ccaller_DiagLv1 ==
  diagFaultActive : Inport
  diagStartUpComp : Inport  Port=2
  diagReset : Inport  Port=3
  diagEnable : Inport  Port=4
  diagDbncEnable : Inport  Port=5
  diagFaultCntThresh : Inport  Port=6
  diagPassCntThresh : Inport  Port=7
  diagUpCnt : Inport  Port=8
  diagDnCnt : Inport  Port=9
  diagHealEn : Inport  Port=10
  DiagDebounceLv1_CCaller : CCaller  FunctionName=DiagDebounceLv1  PortSpecificationStruct="%)30     .    <!<   8    (     @         %    \"     T    !     0         %  0 \"0    $    _    07)G3F%M90  4&]R=$YA;64 4V-O<&4     26YD97@     5'EP90      4VEZ90      27-';&]B86P   X   !     !@    @    $          4    (     0   !     !         !     0    9&EA9T9A=6QT0V]U;G1E<@X   !     !@    @    $          4    (     0   !     !         !     0    9&EA9T9A=6QT0V]U;G1E<@X   !     !@    @    $     ...(+7711 chars)"
  Unit Delay : UnitDelay  SampleTime=-1  HasFrameUpgradeWarning=on
      settings: AttributesFormatString=%<InitialCondition>
  Unit Delay1 : UnitDelay  InitialCondition=uint8(32)  SampleTime=-1  HasFrameUpgradeWarning=on
      settings: AttributesFormatString=%<InitialCondition>
  Unit Delay2 : UnitDelay  InitialCondition=false  SampleTime=-1  HasFrameUpgradeWarning=on
      settings: AttributesFormatString=%<InitialCondition>
  diagFaultStatus : Outport  VectorParamsAs1DForOutWhenUnconnected=off
  diagFaultCnt : Outport  Port=2  VectorParamsAs1DForOutWhenUnconnected=off
  wires:
  DiagDebounceLv1_CCaller/1 -> diagFaultCnt/1, Unit Delay/1
  Unit Delay2/1 -> DiagDebounceLv1_CCaller/3
  DiagDebounceLv1_CCaller/3 -> Unit Delay2/1
  Unit Delay1/1 -> DiagDebounceLv1_CCaller/2
  Unit Delay/1 -> DiagDebounceLv1_CCaller/1
  DiagDebounceLv1_CCaller/2 -> Unit Delay1/1, diagFaultStatus/1
  diagPassCntThresh/1 -> DiagDebounceLv1_CCaller/10
  diagDbncEnable/1 -> DiagDebounceLv1_CCaller/8
  diagEnable/1 -> DiagDebounceLv1_CCaller/7
  diagHealEn/1 -> DiagDebounceLv1_CCaller/13
  diagFaultActive/1 -> DiagDebounceLv1_CCaller/4
  diagFaultCntThresh/1 -> DiagDebounceLv1_CCaller/9
  diagReset/1 -> DiagDebounceLv1_CCaller/6
  diagDnCnt/1 -> DiagDebounceLv1_CCaller/12
  diagStartUpComp/1 -> DiagDebounceLv1_CCaller/5
  diagUpCnt/1 -> DiagDebounceLv1_CCaller/11

== system common_lib/Diagnostics/DTNA_Diag/S_Diag/DiagFaultCounter ==
  diagFaultActive : Inport
  diagStartUpComp : Inport  Port=2
  diagReset : Inport  Port=3
  diagEnable : Inport  Port=4
  diagDbncEnab : Inport  Port=5
  diagFaultCntThresh : Inport  Port=6
  diagPassCntThresh : Inport  Port=7
  diagUpCnt : Inport  Port=8
  diagDnCnt : Inport  Port=9
  diagHealEn : Inport  Port=10
  DiagFaulCounter : Stateflow chart  TreatAsAtomicUnit=on
  diagFaultStatus : Outport  OutputWhenDisabled=reset  InitialOutput=Dem_EventStatusType.DEM_EVENT_STATUS_INIT  VectorParamsAs1DForOutWhenUnconnected=off
  diagFaultCnt : Outport  Port=2  OutputWhenDisabled=reset  InitialOutput=Dem_EventStatusType.DEM_EVENT_STATUS_INIT  VectorParamsAs1DForOutWhenUnconnected=off
  wires:
  diagHealEn/1 -> DiagFaulCounter/10(diagHealEn)
  diagPassCntThresh/1 -> DiagFaulCounter/7(diagPassCntThresh)
  diagStartUpComp/1 -> DiagFaulCounter/2(diagStartUpComp)
  diagDbncEnab/1 -> DiagFaulCounter/5(diagDbncEnab)
  DiagFaulCounter/1(diagFaultStatus) -> diagFaultStatus/1
  diagEnable/1 -> DiagFaulCounter/4(diagEnable)
  diagDnCnt/1 -> DiagFaulCounter/9(diagDnCnt)
  diagUpCnt/1 -> DiagFaulCounter/8(diagUpCnt)
  diagReset/1 -> DiagFaulCounter/3(diagReset)
  diagFaultCntThresh/1 -> DiagFaulCounter/6(diagFaultCntThresh)
  diagFaultActive/1 -> DiagFaulCounter/1(diagFaultActive)
  DiagFaulCounter/2(diagFaultCnt) -> diagFaultCnt/1

== system common_lib/OS/Scheduler with Init/Init Relay/Function Call ==
  InitActive : EnablePort  StatesWhenEnabling=reset  ZeroCross=off
  Function-Call Generator : simulink/Ports & Subsystems/Function-Call Generator  sample_time=-1  numberOfIterations=1
  Init : Outport  VectorParamsAs1DForOutWhenUnconnected=off
  wires:
  Function-Call Generator/1 -> Init/1

== system common_lib/Signal Generators/Signal Generator Components/TestSignalRamp/TestSignalRampEnabled ==
  TestSignalFrequencyIn : Inport
  TestSignalFreqRampEnd : Inport  Port=2
  TestSignalFreqRampTime : Inport  Port=3
  TestSignalReset : Inport  Port=4
  Enable : EnablePort  StatesWhenEnabling=reset  ZeroCross=off
  Ramp : $bdroot/Ctrl/Ramp  TimeStep=TimeStep
  TestSignalFrequency : Outport  VectorParamsAs1DForOutWhenUnconnected=off
  wires:
  Ramp/1 -> TestSignalFrequency/1
  TestSignalReset/1 -> Ramp/4
  TestSignalFreqRampTime/1 -> Ramp/3
  TestSignalFreqRampEnd/1 -> Ramp/2
  TestSignalFrequencyIn/1 -> Ramp/1
